simulink model "backstepping"  (R2021b)
settings: Solver=VariableStepAuto  StartTime=0.0  StopTime=60  RelTol=1e-3
libraries: simulink x1
settings Model: Creator=84232  LastModifiedBy=84232

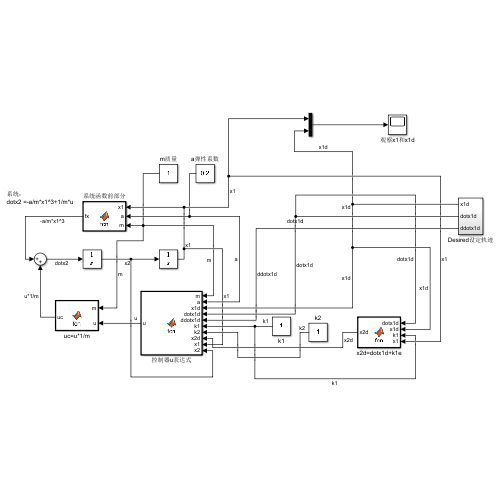
[thumbnail: Simulink's stored preview of the top-level diagram]
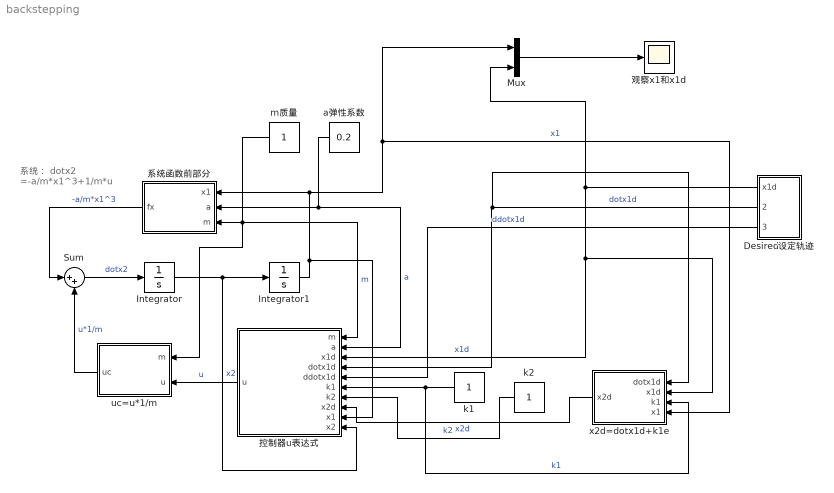
== system backstepping ==
  note: 系统：
      | dotx2 =-a/m*x1^3+1/m*u
  Desired设定轨迹 : Subsystem
  Integrator : Integrator
  Integrator1 : Integrator
  Mux : Mux  Inputs=2
  Sum : Sum  Inputs=|++
  a弹性系数 : Constant  Value=0.2
  k1 : Constant
  k2 : Constant
  m质量 : Constant
  uc=u*1/m : MATLAB Function  TreatAsAtomicUnit=on
  x2d=dotx1d+k1e : MATLAB Function  TreatAsAtomicUnit=on
  控制器u表达式 : MATLAB Function  TreatAsAtomicUnit=on
  系统函数前部分 : MATLAB Function  TreatAsAtomicUnit=on
  观察x1和x1d : Scope
  wires:
  Integrator/1 -> 控制器u表达式/10(x2), Integrator1/1  "x2"
  Integrator1/1 -> 控制器u表达式/9(x1), Mux/1, x2d=dotx1d+k1e/4(x1), 系统函数前部分/1(x1)  "x1"
  Sum/1 -> Integrator/1  "dotx2"
  uc=u*1/m/1(uc) -> Sum/2  "u*1/m"
  系统函数前部分/1(fx) -> Sum/1  "-a/m*x1^3"
  m质量/1 -> 控制器u表达式/1(m), uc=u*1/m/1(m), 系统函数前部分/3(m)  "m"
  a弹性系数/1 -> 控制器u表达式/2(a), 系统函数前部分/2(a)  "a"
  控制器u表达式/1(u) -> uc=u*1/m/2(u)  "u"
  Desired设定轨迹/1(x1d) -> x2d=dotx1d+k1e/2(x1d), 控制器u表达式/3(x1d), Mux/2  "x1d"
  Desired设定轨迹/2(dotx1d) -> 控制器u表达式/4(dotx1d), x2d=dotx1d+k1e/1(dotx1d)  "dotx1d"
  Desired设定轨迹/3(ddotx1d) -> 控制器u表达式/5(ddotx1d)  "ddotx1d"
  k1/1 -> x2d=dotx1d+k1e/3(k1), 控制器u表达式/6(k1)  "k1"
  k2/1 -> 控制器u表达式/7(k2)  "k2"
  x2d=dotx1d+k1e/1(x2d) -> 控制器u表达式/8(x2d)  "x2d"
  Mux/1 -> 观察x1和x1d/1

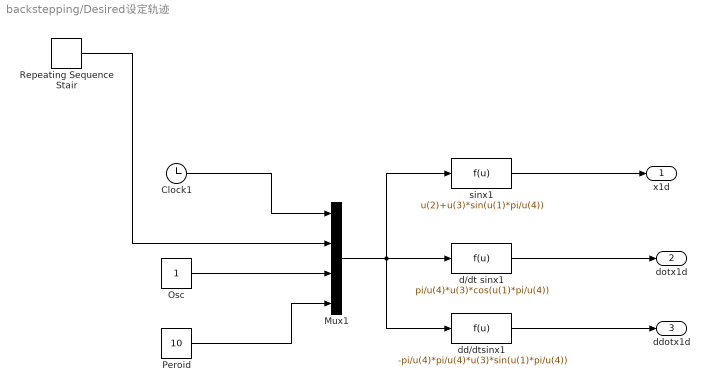
== system backstepping/Desired设定轨迹 ==
  Clock1 : Clock
      settings: Decimation=100
  Mux1 : Mux
  Osc : Constant
  Peroid : Constant  Value=10
  Repeating Sequence Stair : simulink/Sources/Repeating Sequence Stair  OutValues=[1].'  tsamp=10  OutMin=[]  OutMax=[]  OutDataTypeStr=double  OutputDataTypeScalingMode=double  OutDataType=fixdt(0,8)  ConRadixGroup=Best Precision: Vector-wise  OutScaling=2^-12
  d/dt sinx1 : Fcn  Expr=pi/u(4)*u(3)*cos(u(1)*pi/u(4))
  dd/dtsinx1 : Fcn  Expr=-pi/u(4)*pi/u(4)*u(3)*sin(u(1)*pi/u(4))
  sinx1 : Fcn  Expr=u(2)+u(3)*sin(u(1)*pi/u(4))
  x1d : Outport
  dotx1d : Outport  Port=2
  ddotx1d : Outport  Port=3
  wires:
  Repeating Sequence Stair/1 -> Mux1/2
  Clock1/1 -> Mux1/1
  Mux1/1 -> sinx1/1, dd/dtsinx1/1, d/dt sinx1/1
  Osc/1 -> Mux1/3
  Peroid/1 -> Mux1/4
  d/dt sinx1/1 -> dotx1d/1
  dd/dtsinx1/1 -> ddotx1d/1
  sinx1/1 -> x1d/1

== matlab function backstepping/uc=u*1//m ==
  data: m input; u input; uc output
function uc = fcn(m,u)


uc=1\m*u;

== matlab function backstepping/系统函数前部分 ==
  data: x1 input; fx output; a input; m input
function fx = fcn(x1,a,m)


fx = -a/m*x1*x1*x1;

== matlab function backstepping/控制器u表达式 ==
  data: m input; a input; u output; x1d input; dotx1d input; ddotx1d input; k1 input; k2 input; x2d input; x1 input; x2 input
function u = fcn(m,a,x1d,dotx1d,ddotx1d,k1,k2,x2d,x1,x2)

t1=m*(x1d-x1)
t2=m*ddotx1d
t3=m*k1*(dotx1d-x2)
t4=a*x1*x1*x1
t5=m*k2*(x2d-x2)

u=t1+t2+t3+t4+t5

== matlab function backstepping/x2d=dotx1d+k1e ==
  data: dotx1d input; x1d input; x2d output; k1 input; x1 input
function x2d = fcn(dotx1d,x1d,k1,x1)


x2d=dotx1d+k1*(x1d-x1);
